simulink model "backstepping_control"  (R2017a)
settings: Solver=VariableStepAuto  StartTime=0.0  StopTime=tf  RelTol=1e-3
undefined symbols (not defined in the file or in its folder): controlfun, plantfun, x0
settings Model: Creator=bruno  LastModifiedBy=bruno

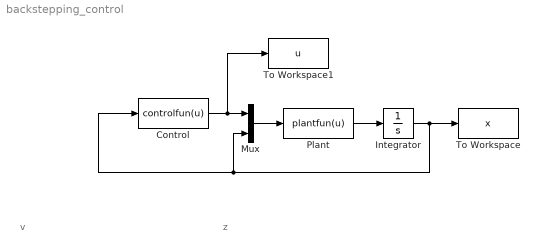
== system backstepping_control ==
  note: z
  note: v
  "Control " : MATLABFcn  MATLABFcn=controlfun(u)  OutputSignalType=real
  Integrator : Integrator  InitialCondition=x0
  Mux : Mux  Inputs=2
  Plant : MATLABFcn  MATLABFcn=plantfun(u)  OutputSignalType=real
  To Workspace : ToWorkspace  VariableName=x  SaveFormat=Timeseries  SampleTime=-1
  To Workspace1 : ToWorkspace  VariableName=u  SaveFormat=Timeseries  SampleTime=-1
  wires:
  Plant/1 -> Integrator/1
  Mux/1 -> Plant/1
  "Control "/1 -> To Workspace1/1, Mux/1
  Integrator/1 -> "Control "/1, Mux/2, To Workspace/1
